simulink model "ControleSimuladoPeixeTesteDiscrizado_R2024a"  (R2024a)
settings: Solver=VariableStepAuto  StartTime=0.0  StopTime=200  RelTol=1e-3
undefined symbols (not defined in the file): Peixe, Ufinal1, Ufinal1Disc
settings Model: Creator=carlo  LastModifiedBy=tynam

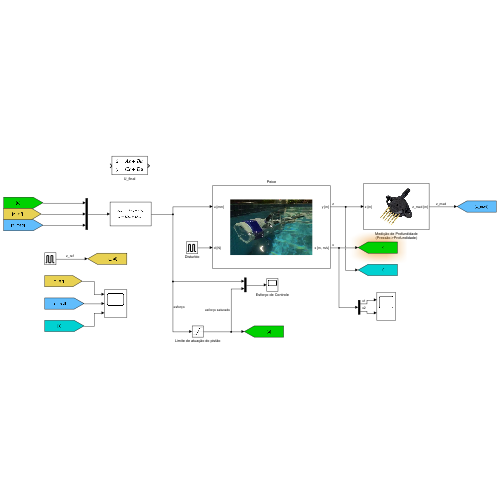
[thumbnail: Simulink's stored preview of the top-level diagram]
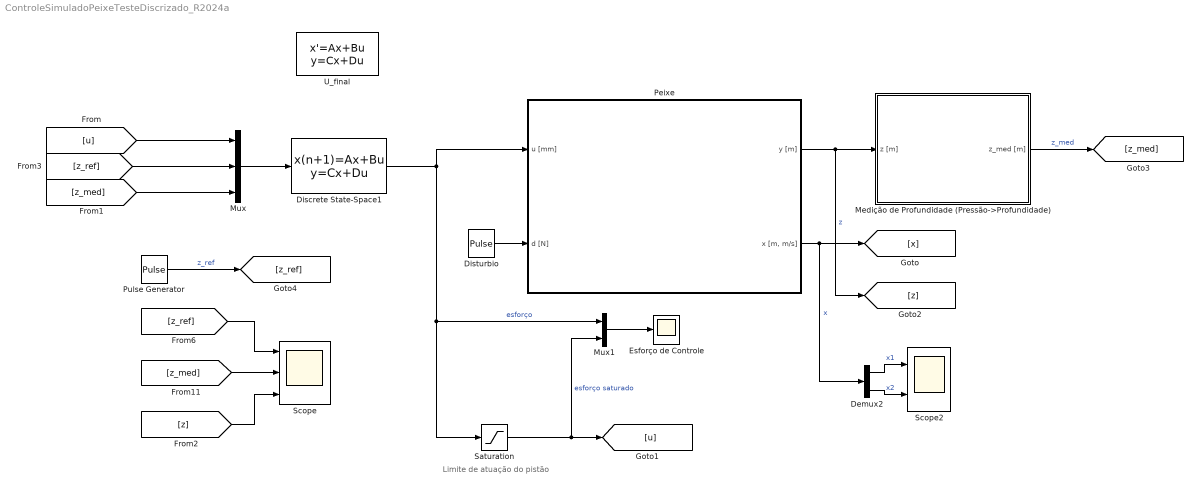
== system ControleSimuladoPeixeTesteDiscrizado_R2024a ==
  note: Limite de atuação do pistão
  Demux2 : Demux  Outputs=2
  Discrete State-Space1 : DiscreteStateSpace  A=Ufinal1Disc.A  B=Ufinal1Disc.B  C=Ufinal1Disc.C  D=Ufinal1Disc.D  SampleTime=0.1
  Disturbio : DiscretePulseGenerator  PulseType=Time based  Amplitude=0.01  Period=240  PulseWidth=50  PhaseDelay=135
  Esforço de Controle : Scope
  Medição de Profundidade (Pressão->Profundidade) : Subsystem
      mask Display: image('mpx5700ap.jpg', [0,0,0,0,80,80]);
  Mux : Mux  Inputs=3
  Mux1 : Mux  Inputs=2
  Peixe : Subsystem
      mask Display: image('peixe_foto.png', [0,0,0,0,70,70]);
  Pulse Generator : DiscretePulseGenerator  PulseType=Time based  Period=100  PulseWidth=50
  Saturation : Saturate  UpperLimit=0.05  LowerLimit=-0.05
  Scope : Scope  NumInputPorts=3
  Scope2 : Scope  NumInputPorts=2
  U_final : StateSpace  A=Ufinal1.A  B=Ufinal1.B  C=Ufinal1.C  D=Ufinal1.D  InitialCondition=0
  wires:
  Pulse Generator/1 -> [z_ref]  "z_ref"
  Peixe/2("x [m, m/s]") -> Demux2/1, [x]  "x"
  Peixe/1(y [m]) -> Medição de Profundidade (Pressão->Profundidade)/1(z [m]), [z]  "z"
  Medição de Profundidade (Pressão->Profundidade)/1(z_med [m]) -> [z_med]  "z_med"
  [z] -> Scope/3
  [z_ref] -> Scope/1
  [z_med] -> Scope/2
  Disturbio/1 -> Peixe/2(d [N])
  Demux2/1 -> Scope2/1  "x1"
  Demux2/2 -> Scope2/2  "x2"
  Saturation/1 -> Mux1/2, [u]  "esforço saturado"
  [u] -> Mux/1
  Mux/1 -> Discrete State-Space1/1
  [z_ref] -> Mux/2
  [z_med] -> Mux/3
  Discrete State-Space1/1 -> Saturation/1, Mux1/1, Peixe/1(u [mm])  "esforço"
  Mux1/1 -> Esforço de Controle/1

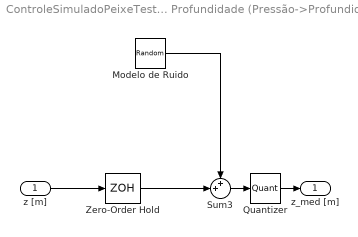
== system ControleSimuladoPeixeTesteDiscrizado_R2024a/Medição de Profundidade (Pressão->Profundidade) ==
  z [m] : Inport
  Modelo de Ruido : RandomNumber  Variance=1e-3  SampleTime=1/200
  Quantizer : Quantizer  QuantizationInterval=0.0081
  Sum3 : Sum  Inputs=++|
  Zero-Order Hold : ZeroOrderHold  SampleTime=1/200
  z_med [m] : Outport
  wires:
  Sum3/1 -> Quantizer/1
  Modelo de Ruido/1 -> Sum3/1
  Zero-Order Hold/1 -> Sum3/2
  z [m]/1 -> Zero-Order Hold/1
  Quantizer/1 -> z_med [m]/1

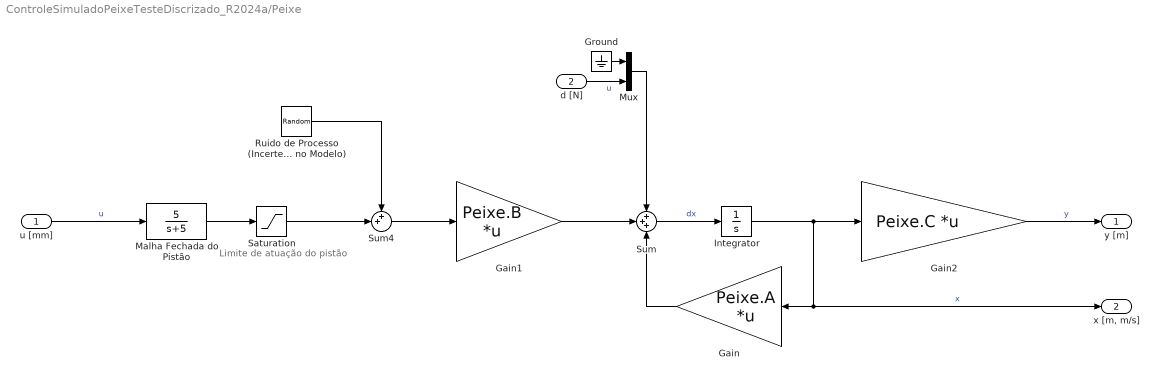
== system ControleSimuladoPeixeTesteDiscrizado_R2024a/Peixe ==
  note: Limite de atuação do pistão
  u [mm] : Inport
  d [N] : Inport  Port=2
  Gain : Gain  Gain=Peixe.A  Multiplication=Matrix(K*u) (u vector)
  Gain1 : Gain  Gain=Peixe.B  Multiplication=Matrix(K*u) (u vector)
  Gain2 : Gain  Gain=Peixe.C  Multiplication=Matrix(K*u) (u vector)
  Ground : Ground
  Integrator : Integrator
  Malha Fechada do Pistão : TransferFcn  Numerator=[5]  Denominator=[1 5]
  Mux : Mux  Inputs=2
  Ruido de Processo (Incertezas no Modelo) : RandomNumber  Variance=0.001*0  SampleTime=0.1
  Saturation : Saturate  UpperLimit=0.05  LowerLimit=-0.05
  Sum : Sum  Inputs=+++
  Sum4 : Sum  Inputs=++|
  y [m] : Outport
  "x [m, m/s]" : Outport  Port=2
  wires:
  Gain/1 -> Sum/3
  Integrator/1 -> Gain2/1, "x [m, m/s]"/1, Gain/1  "x"
  Gain1/1 -> Sum/2
  Gain2/1 -> y [m]/1  "y"
  Sum/1 -> Integrator/1  "dx"
  u [mm]/1 -> Malha Fechada do Pistão/1  "u"
  Sum4/1 -> Gain1/1
  Ruido de Processo (Incertezas no Modelo)/1 -> Sum4/1
  Saturation/1 -> Sum4/2
  Malha Fechada do Pistão/1 -> Saturation/1
  d [N]/1 -> Mux/2  "u"
  Ground/1 -> Mux/1
  Mux/1 -> Sum/1
